simulink model "observateur_sliding_mode_commande_lin"  (R2020a)
settings: Solver=VariableStepAuto  StartTime=0.0  StopTime=10  RelTol=1e-3
undefined symbols (not defined in the file): a, b, K, L_sliding_back
settings Model: Creator=lenovo  LastModifiedBy=lenovo
settings SolverCC: ZeroCrossAlgorithm=Adaptive
settings DebuggingCC: IgnoredZcDiagnostic=none

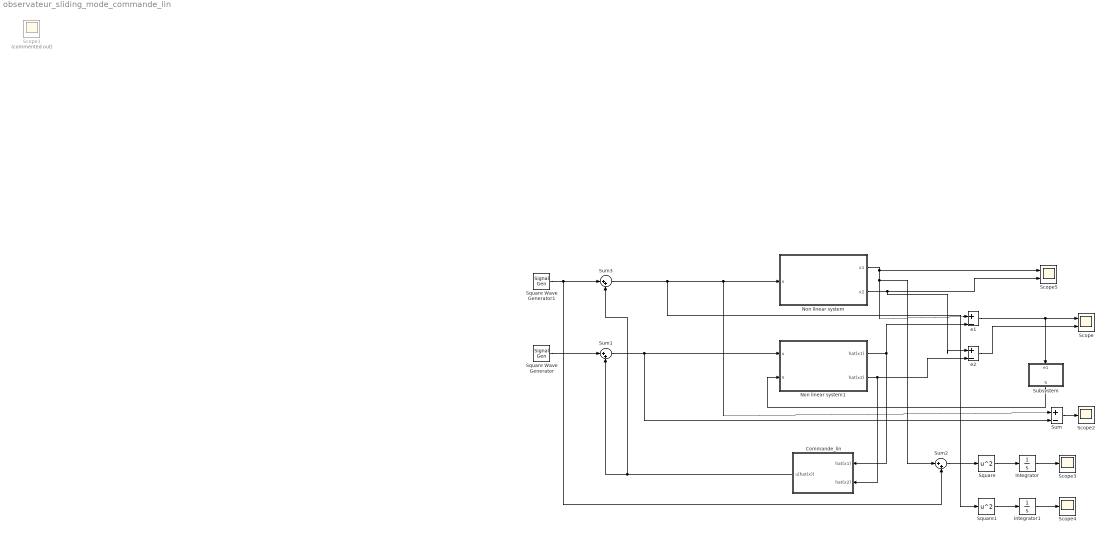
== system observateur_sliding_mode_commande_lin ==
  Commande_lin : Subsystem
  Integrator : Integrator
  Integrator1 : Integrator
  Non linear system : Subsystem
  Non linear system1 : Subsystem
  Scope : Scope  NumInputPorts=2
  Scope1 : Scope  Commented=on
  Scope2 : Scope
  Scope3 : Scope
  Scope4 : Scope
  Scope5 : Scope  NumInputPorts=2
  Square : Math  Operator=square  SaturateOnIntegerOverflow=on
  Square Wave Generator : SignalGenerator  WaveForm=square  Units=rad/sec
  Square Wave Generator1 : SignalGenerator  WaveForm=square  Units=rad/sec
  Square1 : Math  Operator=square  SaturateOnIntegerOverflow=on
  Subsystem : Subsystem
  Sum : Sum  Inputs=|+-
  Sum1 : Sum  Inputs=|++
  Sum2 : Sum  Inputs=|++
  Sum3 : Sum  Inputs=|++
  e1 : Sum  Inputs=|+-
  e2 : Sum  Inputs=|+-
  wires:
  Non linear system/2(x2) -> Scope5/2, e2/1
  e2/1 -> Scope/2
  Sum1/1 -> Sum/2, Non linear system1/1(u)
  Non linear system1/2(hat(x2)) -> Commande_lin/2(hat(x2)), e2/2
  Non linear system1/1(hat(x1)) -> Commande_lin/1(hat(x1)), e1/2
  Square Wave Generator1/1 -> Sum2/2, Sum3/1
  e1/1 -> Subsystem/1(e1), Scope/1
  Non linear system/1(x1) -> Sum2/1, e1/1, Scope5/1
  Square Wave Generator/1 -> Sum1/1
  Subsystem/1(S) -> Non linear system1/2(S)
  Commande_lin/1(u(hat(x))) -> Sum3/2, Sum1/2
  Sum/1 -> Scope2/1
  Sum2/1 -> Square/1
  Sum3/1 -> Square1/1, Sum/1, Non linear system/1(u)
  Integrator1/1 -> Scope4/1
  Square/1 -> Integrator/1
  Integrator/1 -> Scope3/1
  Square1/1 -> Integrator1/1

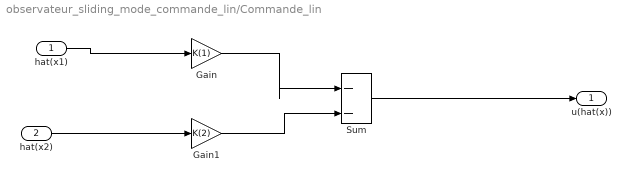
== system observateur_sliding_mode_commande_lin/Commande_lin ==
  hat(x1) : Inport
  hat(x2) : Inport  Port=2
  Gain : Gain  Gain=K(1)
  Gain1 : Gain  Gain=K(2)
  Sum : Sum  Inputs=|--
  u(hat(x)) : Outport
  wires:
  Sum/1 -> u(hat(x))/1
  hat(x2)/1 -> Gain1/1
  Gain/1 -> Sum/1
  hat(x1)/1 -> Gain/1
  Gain1/1 -> Sum/2

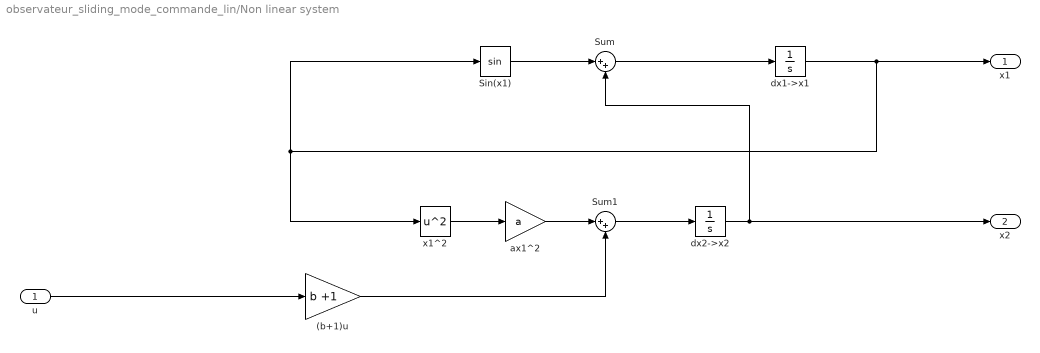
== system observateur_sliding_mode_commande_lin/Non linear system ==
  u : Inport
  (b+1)u : Gain  Gain=b +1
  Sin(x1) : Trigonometry
  Sum : Sum  Inputs=|++
  Sum1 : Sum  Inputs=|++
  ax1^2 : Gain  Gain=a
  dx1->x1 : Integrator
  dx2->x2 : Integrator
  x1^2 : Math  Operator=square  SaturateOnIntegerOverflow=on
  x1 : Outport
  x2 : Outport  Port=2
  wires:
  (b+1)u/1 -> Sum1/2
  dx2->x2/1 -> x2/1, Sum/2
  u/1 -> (b+1)u/1
  ax1^2/1 -> Sum1/1
  dx1->x1/1 -> Sin(x1)/1, x1^2/1, x1/1
  Sin(x1)/1 -> Sum/1
  x1^2/1 -> ax1^2/1
  Sum1/1 -> dx2->x2/1
  Sum/1 -> dx1->x1/1

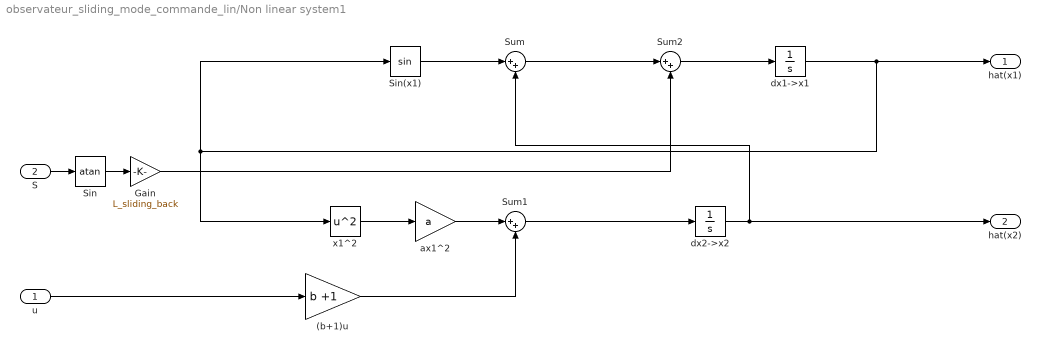
== system observateur_sliding_mode_commande_lin/Non linear system1 ==
  u : Inport
  S : Inport  Port=2
  (b+1)u : Gain  Gain=b +1
  Gain : Gain  Gain=L_sliding_back
  Sin : Trigonometry  Operator=atan
  Sin(x1) : Trigonometry
  Sum : Sum  Inputs=|++
  Sum1 : Sum  Inputs=|++
  Sum2 : Sum  Inputs=|++
  ax1^2 : Gain  Gain=a
  dx1->x1 : Integrator  InitialCondition=1
  dx2->x2 : Integrator  InitialCondition=1
  x1^2 : Math  Operator=square  SaturateOnIntegerOverflow=on
  hat(x1) : Outport
  hat(x2) : Outport  Port=2
  wires:
  (b+1)u/1 -> Sum1/2
  dx2->x2/1 -> hat(x2)/1, Sum/2
  u/1 -> (b+1)u/1
  ax1^2/1 -> Sum1/1
  dx1->x1/1 -> Sin(x1)/1, x1^2/1, hat(x1)/1
  Sin(x1)/1 -> Sum/1
  x1^2/1 -> ax1^2/1
  Sum1/1 -> dx2->x2/1
  Sum2/1 -> dx1->x1/1
  S/1 -> Sin/1
  Sin/1 -> Gain/1
  Gain/1 -> Sum2/2
  Sum/1 -> Sum2/1

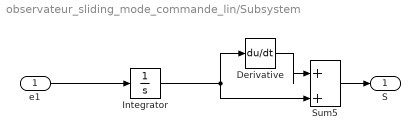
== system observateur_sliding_mode_commande_lin/Subsystem ==
  e1 : Inport
  Derivative : Derivative
  Integrator : Integrator
  Sum5 : Sum  Inputs=|++
  S : Outport
  wires:
  Derivative/1 -> Sum5/1
  Sum5/1 -> S/1
  e1/1 -> Integrator/1
  Integrator/1 -> Sum5/2, Derivative/1
